simulink model "motor_mixer_tester"  (R2016a)
settings: Solver=VariableStepAuto  StartTime=0.0  StopTime=10.0  RelTol=1e-3
settings Model: Creator=GusBus  LastModifiedBy=GusBus

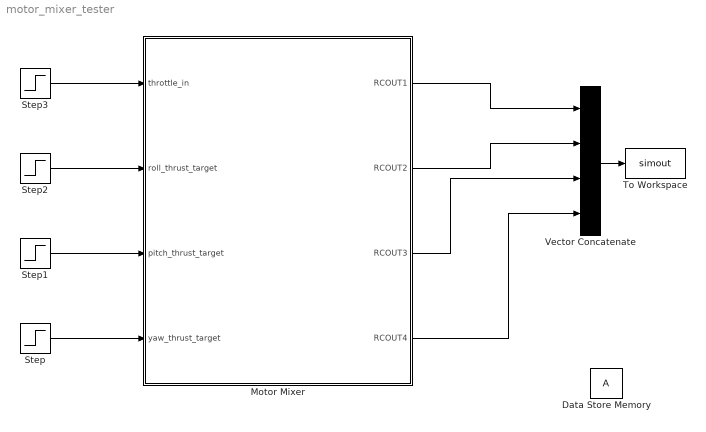
== system motor_mixer_tester ==
  Data Store Memory : DataStoreMemory  ReadBeforeWriteMsg=warning  WriteAfterWriteMsg=warning  WriteAfterReadMsg=warning  ShowAdditionalParam=off
  Motor Mixer : MATLAB Function  TreatAsAtomicUnit=on
  Step{,1..3} (4 alike) : Step  SampleTime=0
  To Workspace : ToWorkspace  VariableName=simout  SaveFormat=Timeseries  SampleTime=-1
  Vector Concatenate : Concatenate  NumInputs=4
  wires:
  Motor Mixer/1(RCOUT1) -> Vector Concatenate/1
  Motor Mixer/2(RCOUT2) -> Vector Concatenate/2
  Motor Mixer/3(RCOUT3) -> Vector Concatenate/3
  Motor Mixer/4(RCOUT4) -> Vector Concatenate/4
  Vector Concatenate/1 -> To Workspace/1
  Step/1 -> Motor Mixer/4(yaw_thrust_target)
  Step1/1 -> Motor Mixer/3(pitch_thrust_target)
  Step2/1 -> Motor Mixer/2(roll_thrust_target)
  Step3/1 -> Motor Mixer/1(throttle_in)

== matlab function motor_mixer_tester/Motor Mixer ==
  data: throttle_in input; roll_thrust_target input; RCOUT1 output; pitch_thrust_target input; yaw_thrust_target input; RCOUT2 output; RCOUT3 output; RCOUT4 output
function [RCOUT1, RCOUT2, RCOUT3, RCOUT4 ]  = motor_mixer(throttle_in, roll_thrust_target, pitch_thrust_target, yaw_thrust_target)
%% Motor Mixer

%
%   Matlab Implementation of the ArduPilot Motor Mixer
%   Outputs Motor Commands based on required rate targets
%
%   
    global pwm_min pwm_max spin_min spin_max thrust_rpyt_out
    % Update throttle filter
    update_throttle_filter(throttle_in);

    % Update battery resistance
    % update_battery_resistance();
                                                                            %For the model, we will always assume we have maximum lift
    % Calc filtered battery voltage and lift_max
    % update_lift_max_from_batt_voltage();

    % Run spool logic
    % output_logic();
    
    % Calculate thrust
    thrust_rpyt_out = output_armed_stabilizing(roll_thrust_target, pitch_thrust_target, yaw_thrust_target);

    % Apply any thrust compensation for the frame
    % thrust_compensation();  %used for tilt rotors and tilt wings
    
    % Convert rpy_thrust values to pwm
    RCOUT1 = pwm_min + (pwm_max-pwm_min)*(spin_min + (spin_max-spin_min)*thrust_rpyt_out(1));
    RCOUT2 = pwm_min + (pwm_max-pwm_min)*(spin_min + (spin_max-spin_min)*thrust_rpyt_out(2));
    RCOUT3 = pwm_min + (pwm_max-pwm_min)*(spin_min + (spin_max-spin_min)*thrust_rpyt_out(3));
    RCOUT4 = pwm_min + (pwm_max-pwm_min)*(spin_min + (spin_max-spin_min)*thrust_rpyt_out(4));
    

end
